simulink model "realtime_test_reference"  (R2025b)
settings: Solver=ode1be  StartTime=0.0  StopTime=1  FixedStep=1/3840  RelTol=1e-3
values from neighbouring files (symbols this model uses):
  load_p = 1e3    (= 1000)    [LG_faults_rework.m]    (also in Small_DataSet.m; Training_Dataset_toolbox_livescript_pipeline_1.m; Training_Dataset_toolbox_livescript_pipeline_2.m; Training_Dataset_toolbox_livescript_pipeline_3.m)
libraries: ee_lib x10, fl_lib x10, nesl_utility x3
settings Model: Creator=faizshaikh  LastModifiedBy=faizshaikh

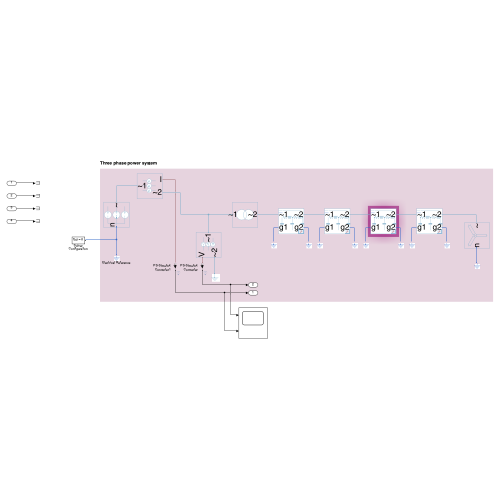
[thumbnail: Simulink's stored preview of the top-level diagram]
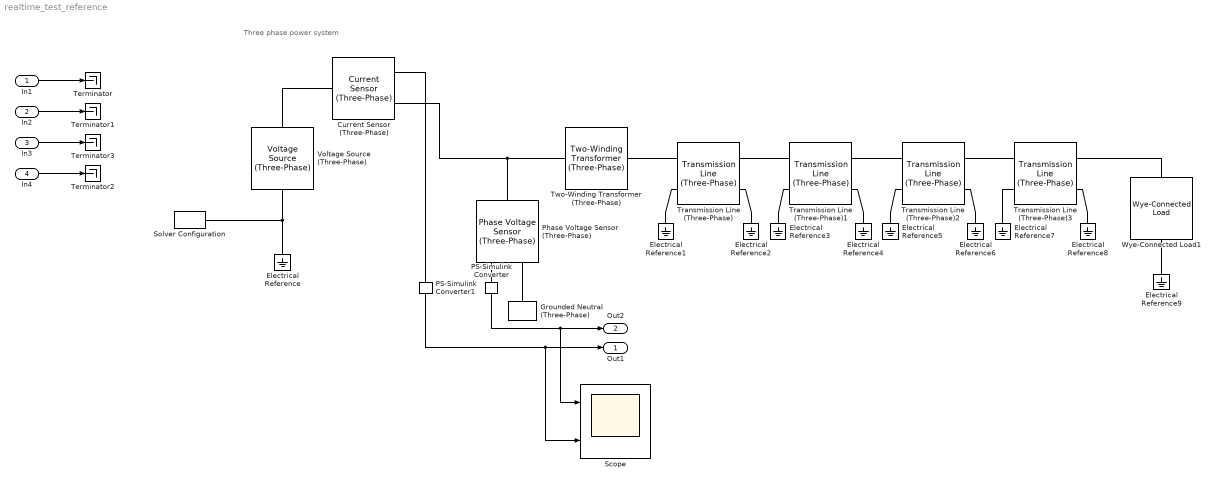
== system realtime_test_reference ==
  note: Three phase power system
  In1 : Inport
  In2 : Inport  Port=2
  In3 : Inport  Port=3
  In4 : Inport  Port=4
  Current Sensor (Three-Phase) : ee_lib/Sensors & Transducers/Current Sensor (Three-Phase)
  Electrical Reference{,1..9} (10 alike) : fl_lib/Electrical/Electrical Elements/Electrical Reference
  Grounded Neutral (Three-Phase) : ee_lib/Connectors & References/Grounded Neutral (Three-Phase)
  PS-Simulink Converter : nesl_utility/PS-Simulink Converter  PhysicalDomain=network_engine_domain  SubClassName=ps_output  LeftPortType=input  RightPortType=output  PseudoPeriodic=off  Frequencies=[]  VectorFormat=inherit  Unit=inherit  AffineConversion=off
  PS-Simulink Converter1 : nesl_utility/PS-Simulink Converter  PhysicalDomain=network_engine_domain  SubClassName=ps_output  LeftPortType=input  RightPortType=output  PseudoPeriodic=off  Frequencies=[]  VectorFormat=inherit  Unit=inherit  AffineConversion=off
  Phase Voltage Sensor (Three-Phase) : ee_lib/Sensors & Transducers/Phase Voltage Sensor (Three-Phase)
  Scope : Scope  NumInputPorts=2
      settings: ActiveDisplayYMinimum=-11492.711091928066  ActiveDisplayYMaximum=19858.774337368995
  Solver Configuration : nesl_utility/Solver Configuration  PhysicalDomain=network_engine_domain  SubClassName=solver  LeftPortType=input  RightPortType=generic  Tones=[]  Harmonics=[]  SimulateNoise=off  Profile=off  UseLocalSampling=off  EnableSwitchedLinearOptims=on  FrequencyDomain=off  UseCCode=off  RelTol=0.001  AbsTol=1e-06  MinStep=1e-09  ToWorkspace=off  RevertToSquareIcSolve=off  NumHomotopyIterations=100  PhasorMode=off  PhasorModeNumHarmonics=1  ConsistencySolver=NEWTON_XTOL_AFTER_FTOL  IndexReductionMethod=DerivativeReplacement  DoDC=off  ResidualTolerance=1e-09  ConsistencyTolSource=GLOBAL  ConsistencyAbsTol=0.001  ConsistencyRelTol=0.001  ConsistencyTolFactor=0.001  UseLocalSolver=off  LocalSolverChoice=NE_BACKWARD_EULER_ADVANCER  ResolveIndetEquations=on  FunctionEvalNumThread=1  LocalSolverSampleTime=0.001  DoFixedCost=off  MaxNonlinIter=3  MaxModeIter=2  ComputeImpulses=off  ImpulseIterations=2  LinearAlgebra=auto  LinearAlgebraNumThread=0  EquationFormulation=NE_TIME_EF  DelaysMemoryBudget=1024  AutomaticFiltering=on  FilteringTimeConstant=0.001  PartitionStorageMethod=AS_NEEDED  PartitionMemoryBudget=1024  PartitionMethod=ROBUST  MultibodyUseLocalSolver=off  MultibodyLocalSolverChoice=ODE1  MultibodyLocalSolverSampleTime=0.001
  Terminator{,1..3} (4 alike) : Terminator
  Transmission Line (Three-Phase) : ee_lib/Passive/Lines/Transmission Line (Three-Phase)  length=100 m  freq=60 Hz  R=0.02 Ohm/km  L=0.5 mH/km  M=0.1 mH/km  Cl=0.3 uF/km  Cg=0.1 uF/km  Rm=0 Ohm/km  ModelTwoSections=ee.enum.enable.yes  N=1  InterfacePosition=interface1 m  N1sec=1  N2sec=1  Access_ground=ee.enum.enable.no  R_parasitic=1e-6 Ohm  G_parasitic=1e-6 1/Ohm
      settings: InternalSimscapePortConfiguration="{\"Bottom\":[],\"Left\":[{\"id\":\"N1\",\"label\":\"~1\",\"type\":\"foundation.electrical.three_phase\"},{\"id\":\"g1\",\"label\":\"g1\",\"type\":\"foundation.electrical.electrical\"}],\"Right\":[{\"id\":\"N2\",\"label\":\"~2\",\"type\":\"foundation.electrical.three_phase\"},{\"id\":\"g2\",\"label\":\"g2\",\"type\":\"foundation.electrical.electrical\"}],\"Top\":[]}"
  Transmission Line (Three-Phase)1 : ee_lib/Passive/Lines/Transmission Line (Three-Phase)  length=100 m  freq=60 Hz  R=0.02 Ohm/km  L=0.5 mH/km  M=0.1 mH/km  Cl=0.3 uF/km  Cg=0.1 uF/km  Rm=0 Ohm/km  ModelTwoSections=ee.enum.enable.yes  N=1  InterfacePosition=interface2 m  N1sec=1  N2sec=1  Access_ground=ee.enum.enable.no  R_parasitic=1e-6 Ohm  G_parasitic=1e-6 1/Ohm
      settings: InternalSimscapePortConfiguration="{\"Bottom\":[],\"Left\":[{\"id\":\"N1\",\"label\":\"~1\",\"type\":\"foundation.electrical.three_phase\"},{\"id\":\"g1\",\"label\":\"g1\",\"type\":\"foundation.electrical.electrical\"}],\"Right\":[{\"id\":\"N2\",\"label\":\"~2\",\"type\":\"foundation.electrical.three_phase\"},{\"id\":\"g2\",\"label\":\"g2\",\"type\":\"foundation.electrical.electrical\"}],\"Top\":[]}"
  Transmission Line (Three-Phase)2 : ee_lib/Passive/Lines/Transmission Line (Three-Phase)  length=100 m  freq=60 Hz  R=0.02 Ohm/km  L=0.5 mH/km  M=0.1 mH/km  Cl=0.3 uF/km  Cg=0.1 uF/km  Rm=0 Ohm/km  ModelTwoSections=ee.enum.enable.yes  N=1  InterfacePosition=interface3 m  N1sec=1  N2sec=1  Access_ground=ee.enum.enable.no  R_parasitic=1e-6 Ohm  G_parasitic=1e-6 1/Ohm
      settings: InternalSimscapePortConfiguration="{\"Bottom\":[],\"Left\":[{\"id\":\"N1\",\"label\":\"~1\",\"type\":\"foundation.electrical.three_phase\"},{\"id\":\"g1\",\"label\":\"g1\",\"type\":\"foundation.electrical.electrical\"}],\"Right\":[{\"id\":\"N2\",\"label\":\"~2\",\"type\":\"foundation.electrical.three_phase\"},{\"id\":\"g2\",\"label\":\"g2\",\"type\":\"foundation.electrical.electrical\"}],\"Top\":[]}"
  Transmission Line (Three-Phase)3 : ee_lib/Passive/Lines/Transmission Line (Three-Phase)  length=100 m  freq=60 Hz  R=0.02 Ohm/km  L=0.5 mH/km  M=0.1 mH/km  Cl=0.3 uF/km  Cg=0.1 uF/km  Rm=0 Ohm/km  ModelTwoSections=ee.enum.enable.yes  N=1  InterfacePosition=interface4 m  N1sec=1  N2sec=1  Access_ground=ee.enum.enable.no  R_parasitic=1e-6 Ohm  G_parasitic=1e-6 1/Ohm
      settings: InternalSimscapePortConfiguration="{\"Bottom\":[],\"Left\":[{\"id\":\"N1\",\"label\":\"~1\",\"type\":\"foundation.electrical.three_phase\"},{\"id\":\"g1\",\"label\":\"g1\",\"type\":\"foundation.electrical.electrical\"}],\"Right\":[{\"id\":\"N2\",\"label\":\"~2\",\"type\":\"foundation.electrical.three_phase\"},{\"id\":\"g2\",\"label\":\"g2\",\"type\":\"foundation.electrical.electrical\"}],\"Top\":[]}"
  Two-Winding Transformer (Three-Phase) : ee_lib/Passive/Transformers/Two-Winding Transformer (Three-Phase)  SRated=100e6 A*V  FRated=60 Hz  Winding1Connection=ee.enum.windingconnection.Yg  VRated1=10 kV  Winding2Connection=ee.enum.windingconnection.Yg  VRated2=400 V  CoreType=ee.enum.coretype.threelimb  pu_Rw1=0.01  pu_Rw2=0.01  leakage_reactance_option=ee.enum.transformer_leakage.exclude  pu_Xl1=0.05  pu_Xl2=0.05  magnetizing_resistance_option=ee.enum.transformer_magnetizingResistance.exclude  pu_Rm=500  magnetizing_reactance_option=ee.enum.transformer_magnetizingReactance.exclude  saturation_option=ee.enum.transformer_saturation.exclude  pu_Xm=500  current_data=[0, .002, 1, 2]  magnetic_flux_data=[0, 1.2, 1.5, 1.51]  pu_X0=0.5  i1_specify=off  i1_priority=None  i1=[0, 0, 0] A  i1_nominal_specify=off  i1_nominal_value=1  i1_nominal_unit=A  i2_specify=off  i2_priority=None  i2=[0, 0, 0] A  i2_nominal_specify=off  i2_nominal_value=1  i2_nominal_unit=A  phi_specify=off  phi_priority=None  phi=[0, 0, 0]  phi_nominal_specify=off  phi_nominal_value=1  phi_nominal_unit=1  power_dissipated_specify=off  power_dissipated_priority=None  power_dissipated=0 W  power_dissipated_nominal_specify=off  power_dissipated_nominal_value=1  power_dissipated_nominal_unit=W
      settings: InternalSimscapePortConfiguration="{\"Bottom\":[],\"Left\":[{\"id\":\"N1\",\"label\":\"~1\",\"type\":\"foundation.electrical.three_phase\"}],\"Right\":[{\"id\":\"N2\",\"label\":\"~2\",\"type\":\"foundation.electrical.three_phase\"}],\"Top\":[]}"
  Voltage Source (Three-Phase) : ee_lib/Sources/Voltage Source (Three-Phase)  vline_rms=10 kV  shift=0 deg  freq=60 Hz  impedance_option=1  SShortCircuit=1e6 A*V  XR=15  R=0.01 Ohm  L=3.97e-4 H  harmonic_option=0  harmonic_orders=[5, 7, 11, 13]  harmonic_ratios=[.1, .1, .1, .1]  G_parasitic=0 1/Ohm  I_specify=off  I_priority=None  I=[0, 0, 0] A  I_nominal_specify=off  I_nominal_value=1  I_nominal_unit=A
  Wye-Connected Load1 : ee_lib/Passive/RLC Assemblies/Wye-Connected Load  port_option=ee.enum.threePhasePort.composite  parameterization=ee.enum.rlc.parameterization.ratedpower  component_structure=ee.enum.rlc.structure.R  component_structure_PQ=ee.enum.rlc.structure.R  R=1 Ohm  L=1e-3 H  C=1e-6 F  VRated=24e3 V  FRated=60 Hz  P=load_p W  Qpos=1e2 A*V  Qneg=-1e2 A*V  R_parasitic=0 Ohm  G_parasitic=0 1/Ohm  R_parasitic_PQ=0 Ohm  G_parasitic_PQ=0 1/Ohm  Vmag0=24e3 V  Vang0=0 deg  Freq0=60 Hz  IL_specify=off  IL_priority=High  IL=[0, 0, 0] A  IL_nominal_specify=off  IL_nominal_value=1  IL_nominal_unit=A  VC_specify=off  VC_priority=High  VC=[0, 0, 0] V  VC_nominal_specify=off  VC_nominal_value=1  VC_nominal_unit=V
  Out1 : Outport
  Out2 : Outport  Port=2
  wires:
  PS-Simulink Converter1/1 -> Scope/2, Out1/1
  PS-Simulink Converter/1 -> Scope/1, Out2/1
  In1/1 -> Terminator/1
  In2/1 -> Terminator1/1
  In3/1 -> Terminator3/1
  In4/1 -> Terminator2/1
  connections:
  Phase Voltage Sensor (Three-Phase)/LConn1 -- Current Sensor (Three-Phase)/RConn2 -- Two-Winding Transformer (Three-Phase)/LConn1
  Voltage Source (Three-Phase)/LConn1 -- Solver Configuration/RConn1 -- Electrical Reference/LConn1
  Electrical Reference6/LConn1 -- Transmission Line (Three-Phase)2/RConn2
  Electrical Reference8/LConn1 -- Transmission Line (Three-Phase)3/RConn2
  Electrical Reference2/LConn1 -- Transmission Line (Three-Phase)/RConn2
  Electrical Reference3/LConn1 -- Transmission Line (Three-Phase)1/LConn2
  Transmission Line (Three-Phase)/LConn1 -- Two-Winding Transformer (Three-Phase)/RConn1
  Grounded Neutral (Three-Phase)/LConn1 -- Phase Voltage Sensor (Three-Phase)/RConn2
  Current Sensor (Three-Phase)/RConn1 -- PS-Simulink Converter1/LConn1
  Wye-Connected Load1/RConn1 -- Electrical Reference9/LConn1
  PS-Simulink Converter/LConn1 -- Phase Voltage Sensor (Three-Phase)/RConn1
  Transmission Line (Three-Phase)3/LConn2 -- Electrical Reference7/LConn1
  Wye-Connected Load1/LConn1 -- Transmission Line (Three-Phase)3/RConn1
  Transmission Line (Three-Phase)/RConn1 -- Transmission Line (Three-Phase)1/LConn1
  Voltage Source (Three-Phase)/RConn1 -- Current Sensor (Three-Phase)/LConn1
  Electrical Reference4/LConn1 -- Transmission Line (Three-Phase)1/RConn2
  Electrical Reference1/LConn1 -- Transmission Line (Three-Phase)/LConn2
  Transmission Line (Three-Phase)2/RConn1 -- Transmission Line (Three-Phase)3/LConn1
  Electrical Reference5/LConn1 -- Transmission Line (Three-Phase)2/LConn2
  Transmission Line (Three-Phase)1/RConn1 -- Transmission Line (Three-Phase)2/LConn1
